simulink model "Fahrzeugmodell"  (R2020b)
settings: Solver=VariableStepAuto  StartTime=0.0  StopTime=inf  RelTol=1e-3
values from neighbouring files (symbols this model uses):
  a = 1.25    [Fahrdynamik.m]    (also in ZweiDFahranimation.m = 1.35)
  A_f = 1.6 + 0.00056*(m-765)    (= 1.933088)    [Fahrdynamik.m]
  aa = 0    [Fahrdynamik.m]
  b = []    [Bezier.m]    (also in Bezier1.m; Fahrdynamik.m = 1.35; TestenBezier.m; ZweiDFahranimation.m = 1.35)
  bb = 0.5    [Fahrdynamik.m]
  c1 = 52480    [Fahrdynamik.m]
  c2 = 88416    [Fahrdynamik.m]
  c_w = 0.34    [Fahrdynamik.m]
  f_r = 0.015    [Fahrdynamik.m]
  g = 9.81    [Fahrdynamik.m]
  Iz = 1992.54    [Fahrdynamik.m]
  m = 1359.8    [Fahrdynamik.m]
  roh = 1.225    [Fahrdynamik.m]
undefined symbols (not defined in the file or in its folder): DiscIntNeverNeededParam
libraries: simulink x10, simulink_extras x9, robotmobilelib x3, vrlib x1, sldrtlib x1, autolibshared x1
settings Model: SimulationMode=accelerator  PacingRate=0.100000  Creator=59258  LastModifiedBy=59258
settings SolverCC: AlgebraicLoopSolver=LineSearch
settings RTWCC: GenCodeOnly=on

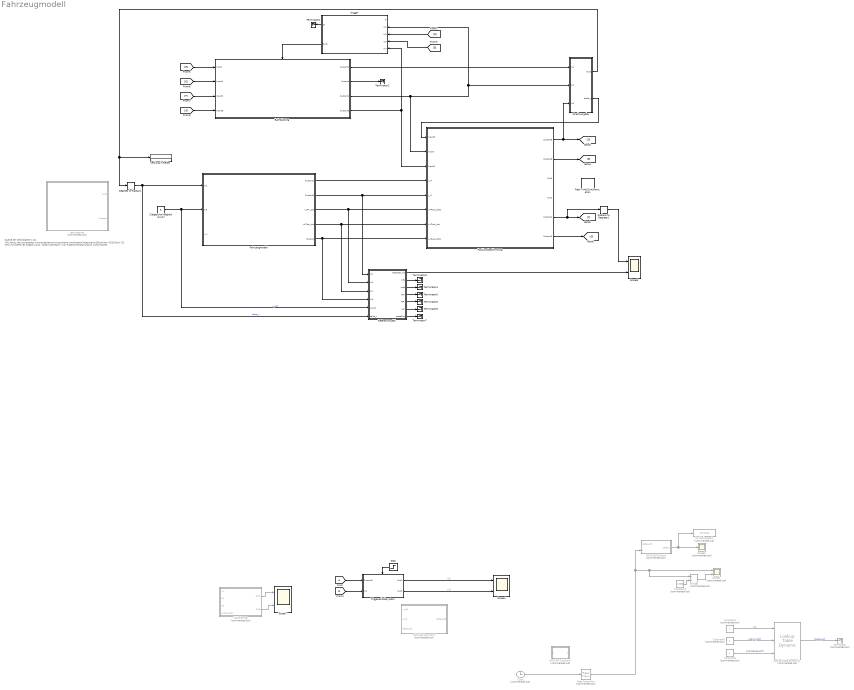
== system Fahrzeugmodell ==
  note: Quelle der Deckblättern:
      | [1] URL:https://en.nissanqatar.com/experience-nissan/news-and-events/latestnews/09-January-2019.html
      | [2] URL:Volvo/SPS
      | [3] Ziegler Julius, {Optimale Bahn- und Trajektorienplanung für Automoblie}
  Bahnplanung : Subsystem  TreatAsAtomicUnit=on  SystemSampleTime=111
      mask Display: image('Deckblatt.png'); % Use "Edit Image" on toolstrip to change.
  Clock : Clock  Commented=on
      settings: Decimation=1000
  Constant3 : Constant  Commented=on  Value=0.066
  Constant4 : Constant  Commented=on
  Constant5 : Constant  Commented=on
  Constant6 : Constant  Commented=on
  Degrees to Radians : simulink_extras/Transformations/Degrees to Radians
  Direktvorgabe : Subsystem
  Divide1 : Product  Commented=on  Inputs=*/
  Fahrzeugmodell : Subsystem  SystemSampleTime=0.5
      settings: MinAlgLoopOccurrences=on
      mask Display: image('Nissan Leaf.jpg'); % Use "Edit Image" on toolstrip to change.
  Kalibrierung : Subsystem  Commented=on  TreatAsAtomicUnit=on  SystemSampleTime=0.01
  Lenkung in Reifen : Display
  Lenkungsrad : Subsystem  Commented=on
  Lookup Table Dynamic1 : simulink/Lookup Tables/Lookup Table Dynamic  Commented=on  LookUpMeth=Use Input Above  OutDataType=fixdt('double')  OutScaling=[]  OutputDataTypeScalingMode=Specify via dialog  OutDataTypeStr=double  RndMeth=Convergent  DoSatur=off
  MATLAB Function : MATLAB Function  Commented=on  TreatAsAtomicUnit=on  SystemSampleTime=0.066
  MATLAB Function1 : MATLAB Function  Commented=on  TreatAsAtomicUnit=on
  MATLAB Function2 : MATLAB Function  Commented=on  TreatAsAtomicUnit=on
  Positionsbestimmung : Subsystem  SystemSampleTime=0.05
      mask Display: image('Volvo-testet-die-magnetische-Positionsbestimmung.jpg'); % Use "Edit Image" on toolstrip to change.
  Radians to Degrees1 : simulink_extras/Transformations/Radians to Degrees
  Rate Transition : RateTransition  Commented=on  OutPortSampleTime=0.066
  Real-Time Synchronization : sldrtlib/Real-Time Synchronization  SampleTime=0.1  MaxMissedTicks=30  ShowMissedTicks=off  YieldWhenWaiting=off
  Referenzmodell : Subsystem
  Scope1 : Scope  Commented=on  NumInputPorts=2
  Scope2 : Scope  Commented=on
  Scope3 : Scope  NumInputPorts=2
  Scope4 : Scope  NumInputPorts=2
  Scope7 : Scope  NumInputPorts=2
  Step : Step  Time=7.7  SampleTime=0
  Terminator : Terminator  Commented=on
  Terminator{1..8} (8 alike) : Terminator
  To Workspace1 : ToWorkspace  Commented=on  VariableName=simout1  SaveFormat=Timeseries  SampleTime=-1
  Trigger : Subsystem
  Triggered Subsystem : Subsystem  TreatAsAtomicUnit=on
  Zielgeschwindigkeit (km/h) : Constant  Value=5
  wires:
  Step/1 -> Triggered Subsystem/Trigger
  Triggered Subsystem/1(Out1) -> Scope4/1  "x_k"
  [A] -> Triggered Subsystem/1(Outport2)
  [B] -> Triggered Subsystem/2(In2)
  Triggered Subsystem/2(Out2) -> Scope4/2  "y_k"
  Kalibrierung/1(Out1) -> Scope7/1
  Kalibrierung/2(Out2) -> Scope7/2
  [F] -> Bahnplanung/3(Inport2)
  [G] -> Bahnplanung/4(Inport3)
  Degrees to Radians/1 -> Fahrzeugmodell/1(In1), Referenzmodell/6(delta_v)  "delta_v"
  Fahrzeugmodell/1(Outport1) -> Positionsbestimmung/4(x_M)
  Fahrzeugmodell/2(Outport2) -> Referenzmodell/1(In2), Positionsbestimmung/5(y_M)
  Fahrzeugmodell/3(x2=y_dot) -> Referenzmodell/2(In3), Positionsbestimmung/6(x4=psi_dot2)
  Positionsbestimmung/6(Outport2) -> [G]
  Bahnplanung/4(Outport3) -> Positionsbestimmung/3(Inport1), Trigger/5(In4)
  Rate Transition/1 -> MATLAB Function/2(t), Divide1/1, Scope1/1
  MATLAB Function/1(delta_v) -> To Workspace1/1, Scope2/1
  Clock/1 -> Rate Transition/1
  Constant3/1 -> Divide1/2
  Divide1/1 -> Scope1/2
  Positionsbestimmung/5(Outport1) -> [F], Radians to Degrees1/1
  Bahnplanung/3(Outport1) -> Trigger/2(In2), Direktvorgabe/2(In2), Positionsbestimmung/2(Inport)
  Radians to Degrees1/1 -> Scope3/1
  Fahrzeugmodell/4(x4=psi_dot) -> Referenzmodell/3(In4), Positionsbestimmung/7(x4=psi_dot)
  Positionsbestimmung/1(Outport5) -> Direktvorgabe/3(In3), [D]
  Positionsbestimmung/2(Outport6) -> [E]
  [D] -> Bahnplanung/1(Inport)
  [E] -> Bahnplanung/2(Inport1)
  Constant4/1 -> Lookup Table Dynamic1/1  "x_s"
  Lookup Table Dynamic1/1 -> Terminator/1  "kappa_soll"
  Constant5/1 -> Lookup Table Dynamic1/2  "Array[x_soll]"
  Constant6/1 -> Lookup Table Dynamic1/3  "Array[kappa_soll]"
  Fahrzeugmodell/5(Outport) -> Referenzmodell/4(In5), Positionsbestimmung/8(x4=psi_dot1)
  Bahnplanung/1(Outport2) -> Direktvorgabe/1(In1)
  Direktvorgabe/1(Out1) -> Degrees to Radians/1, Lenkung in Reifen/1
  Direktvorgabe/2(delta_v) -> Positionsbestimmung/1(Inport2)
  Zielgeschwindigkeit (km/h)/1 -> Referenzmodell/5(Input1), Fahrzeugmodell/2(In3)  "v_soll"
  Trigger/2(Out2) -> Bahnplanung/Enable
  Trigger/1(!Q) -> Terminator1/1
  Bahnplanung/2(Outport) -> Terminator2/1
  Referenzmodell/1(Degrees out) -> Scope3/2
  Referenzmodell/2(Info) -> Terminator3/1
  Referenzmodell/3(xdot) -> Terminator4/1
  Referenzmodell/4(FzF) -> Terminator5/1
  Referenzmodell/5(FzR) -> Terminator6/1
  Referenzmodell/7(stateDot) -> Terminator7/1
  Referenzmodell/6(psi) -> Terminator8/1
  [D] -> Trigger/3(In3)
  [E] -> Trigger/4(In5)

== system Fahrzeugmodell/Bahnplanung ==
  Inport : Inport
  Inport1 : Inport  Port=2
  Inport2 : Inport  Port=3
  Inport3 : Inport  Port=4
  Enable : EnablePort
  Constant : Constant  Value=0  VectorParams1D=off  SampleTime=-1
  Equal : RelationalOperator  Operator===  OutDataTypeStr=boolean  RndMeth=Simplest
  Scope : Scope
  Stop Simulation : Stop  Commented=on
  Subsystem : Subsystem
  Outport2 : Outport
  Outport : Outport  Port=2
  Outport1 : Outport  Port=3
  Outport3 : Outport  Port=4
  wires:
  Inport/1 -> Subsystem/1(Inport)  "x_s"
  Inport1/1 -> Subsystem/2(Inport1)  "y_s"
  Inport2/1 -> Subsystem/3(Inport2)  "psi_s"
  Inport3/1 -> Subsystem/4(Inport3)
  Subsystem/1(Outport1) -> Outport2/1
  Subsystem/2(Outport) -> Equal/1, Outport/1
  Subsystem/3(Outport2) -> Outport1/1
  Subsystem/4(Outport3) -> Outport3/1
  Constant/1 -> Equal/2
  Equal/1 -> Stop Simulation/1, Scope/1

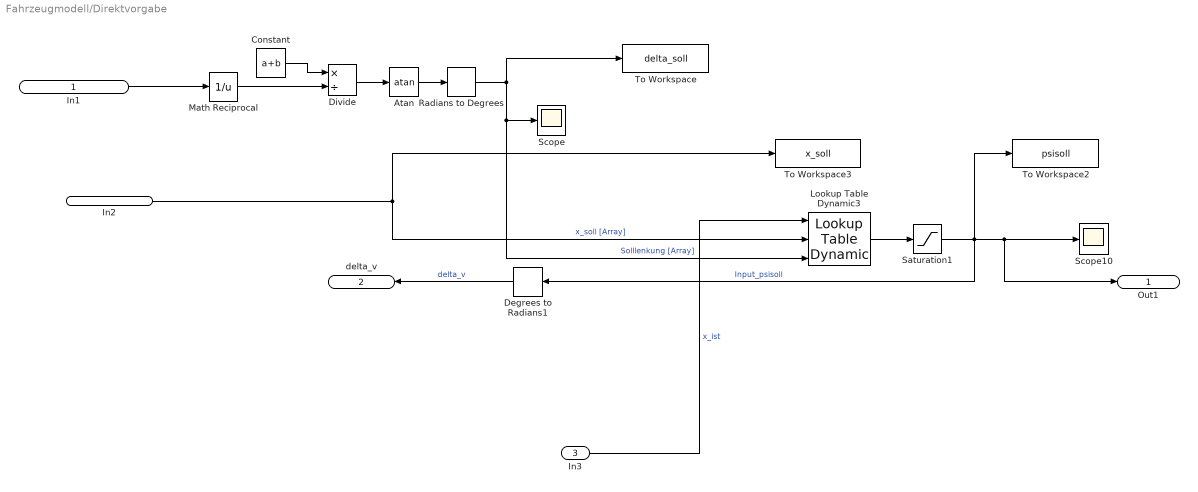
== system Fahrzeugmodell/Direktvorgabe ==
  In1 : Inport
  In2 : Inport  Port=2
  In3 : Inport  Port=3
  Atan : Trigonometry  Operator=atan
  Constant : Constant  Value=a+b
  Degrees to Radians1 : simulink_extras/Transformations/Degrees to Radians
  Divide : Product  Inputs=*/  RndMeth=Zero  SaturateOnIntegerOverflow=on
  Lookup Table Dynamic3 : simulink/Lookup Tables/Lookup Table Dynamic  LookUpMeth=Use Input Nearest  OutDataType=fixdt('double')  OutScaling=[]  OutputDataTypeScalingMode=Specify via dialog  OutDataTypeStr=double  RndMeth=Nearest  DoSatur=off
  Math Reciprocal : Math  Operator=reciprocal  SignedPower=on  SaturateOnIntegerOverflow=on
  Radians to Degrees : simulink_extras/Transformations/Radians to Degrees
  Saturation1 : Saturate  UpperLimit=24.46  LowerLimit=-24.46
  Scope : Scope
  Scope10 : Scope
  To Workspace : ToWorkspace  VariableName=delta_soll  SaveFormat=Timeseries  SampleTime=-1
  To Workspace2 : ToWorkspace  VariableName=psisoll  SaveFormat=Timeseries  SampleTime=-1
  To Workspace3 : ToWorkspace  VariableName=x_soll  SaveFormat=Timeseries  SampleTime=-1
  Out1 : Outport
  delta_v : Outport  Port=2
  wires:
  Math Reciprocal/1 -> Divide/2
  Saturation1/1 -> Degrees to Radians1/1, Out1/1, Scope10/1, To Workspace2/1  "Input_psisoll"
  Atan/1 -> Radians to Degrees/1
  Divide/1 -> Atan/1
  Lookup Table Dynamic3/1 -> Saturation1/1
  Radians to Degrees/1 -> Lookup Table Dynamic3/3, Scope/1, To Workspace/1  "Solllenkung [Array]"
  In3/1 -> Lookup Table Dynamic3/1  "x_ist"
  In2/1 -> Lookup Table Dynamic3/2, To Workspace3/1  "x_soll [Array]"
  Constant/1 -> Divide/1
  In1/1 -> Math Reciprocal/1
  Degrees to Radians1/1 -> delta_v/1  "delta_v"

== system Fahrzeugmodell/Fahrzeugmodell ==
  In1 : Inport
  In3 : Inport  Port=2
  v_x : Inport  Port=3
  Laengsdynamik : Subsystem
  Querdynamik : Subsystem
  Scope : Scope  NumInputPorts=5
  Scope1 : Scope  NumInputPorts=2
  physikalische Koordinate : Subsystem
  Outport1 : Outport
  Outport2 : Outport  Port=2
  x2=y_dot : Outport  Port=3
  x4=psi_dot : Outport  Port=4
  Outport : Outport  Port=5
  wires:
  Querdynamik/2(x2=y_dot) -> Scope/2, x2=y_dot/1, Laengsdynamik/2(Inport)
  Querdynamik/3(x3=psi) -> Scope/3
  Querdynamik/1(x1=y) -> Scope/1
  Querdynamik/5(Outport) -> Scope/5
  Querdynamik/4(x4=psi_dot) -> Laengsdynamik/3(Inport1), x4=psi_dot/1, Scope/4, physikalische Koordinate/2(x4=psi_dot)
  In3/1 -> Laengsdynamik/1(In1)
  physikalische Koordinate/1(x_Koordinate des Modells um Antenne) -> Outport1/1
  In1/1 -> Querdynamik/1(In1)
  physikalische Koordinate/2(Outport2) -> Outport2/1
  Laengsdynamik/2(Out1) -> Scope1/2
  Laengsdynamik/1(v_x) -> Outport/1, Scope1/1, physikalische Koordinate/1(v_x), Querdynamik/2(v_x)

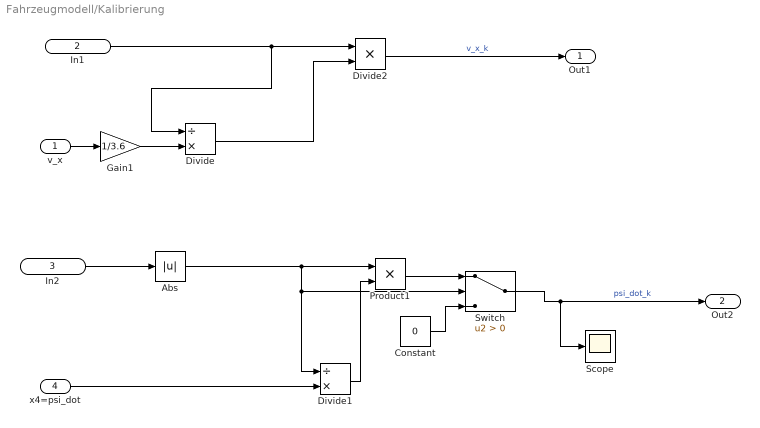
== system Fahrzeugmodell/Kalibrierung ==
  v_x : Inport
  In1 : Inport  Port=2
  In2 : Inport  Port=3
  x4=psi_dot : Inport  Port=4
  Abs : Abs
  Constant : Constant  Value=0
  Divide : Product  Inputs=/*
  Divide1 : Product  Inputs=/*
  Divide2 : Product  Inputs=**
  Gain1 : Gain  Gain=1/3.6
  Product1 : Product
  Scope : Scope
  Switch : Switch  Criteria=u2 > Threshold
  Out1 : Outport
  Out2 : Outport  Port=2
  wires:
  Divide2/1 -> Out1/1  "v_x_k"
  Divide/1 -> Divide2/2
  x4=psi_dot/1 -> Divide1/2
  Product1/1 -> Switch/1
  In2/1 -> Abs/1
  In1/1 -> Divide2/1, Divide/1
  Gain1/1 -> Divide/2
  v_x/1 -> Gain1/1
  Divide1/1 -> Product1/2
  Constant/1 -> Switch/3
  Abs/1 -> Divide1/1, Switch/2, Product1/1
  Switch/1 -> Out2/1, Scope/1  "psi_dot_k"

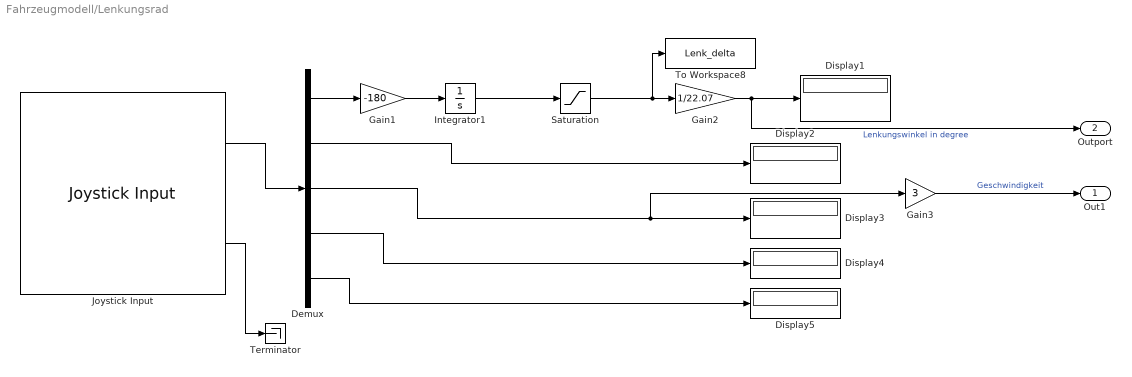
== system Fahrzeugmodell/Lenkungsrad ==
  Demux : Demux  Outputs=5
  Display{1..5} (5 alike) : Display
  Gain1 : Gain  Gain=-180
  Gain2 : Gain  Gain=1/22.07
  Gain3 : Gain  Gain=3
  Integrator1 : Integrator  InitialCondition=0.001
  Joystick Input : vrlib/Joystick Input  joyid=1  adjustports=on  forcefeed=off
  Saturation : Saturate  UpperLimit=540  LowerLimit=-540
  Terminator : Terminator
  To Workspace8 : ToWorkspace  VariableName=Lenk_delta  SaveFormat=Timeseries  SampleTime=-1
  Out1 : Outport
  Outport : Outport  Port=2
  wires:
  Joystick Input/1 -> Demux/1
  Saturation/1 -> To Workspace8/1, Gain2/1
  Gain2/1 -> Outport/1, Display1/1  "Lenkungswinkel in degree"
  Demux/3 -> Gain3/1, Display3/1
  Integrator1/1 -> Saturation/1
  Joystick Input/2 -> Terminator/1
  Demux/2 -> Display2/1
  Demux/1 -> Gain1/1
  Demux/4 -> Display4/1
  Gain1/1 -> Integrator1/1
  Demux/5 -> Display5/1
  Gain3/1 -> Out1/1  "Geschwindigkeit"

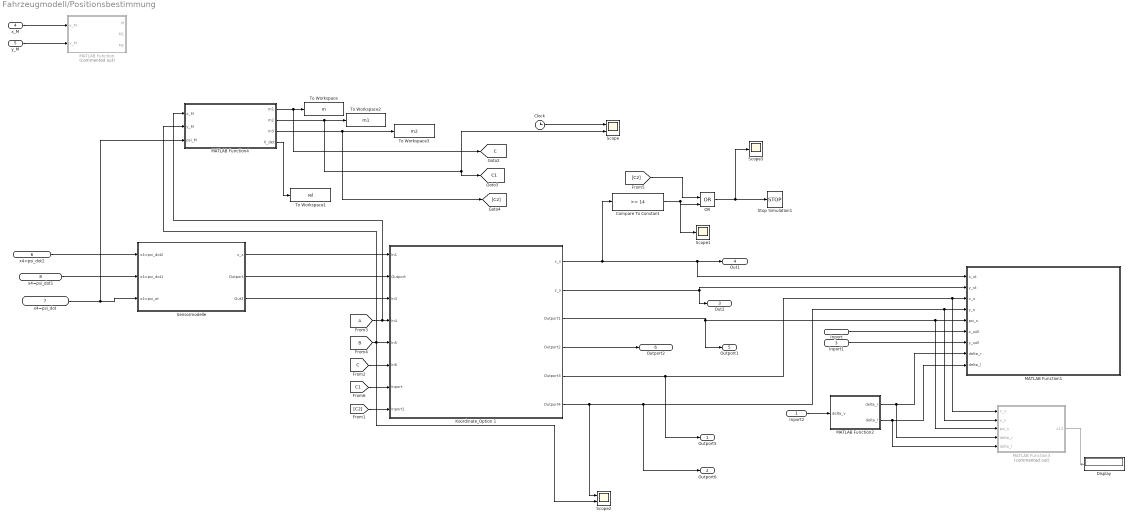
== system Fahrzeugmodell/Positionsbestimmung ==
  Inport2 : Inport
  Inport : Inport  Port=2
  Inport1 : Inport  Port=3
  x_M : Inport  Port=4
  y_M : Inport  Port=5
  x4=psi_dot2 : Inport  Port=6
  x4=psi_dot : Inport  Port=7
  x4=psi_dot1 : Inport  Port=8
  Clock : Clock
  Compare To Constant : simulink/Logic and Bit Operations/Compare To Constant  relop=>=  const=14  OutDataTypeStr=boolean
  Display : Display
  Koordinate_Option 1 : Subsystem
  MATLAB Function : MATLAB Function  Commented=on  TreatAsAtomicUnit=on  SystemSampleTime=0.01
  MATLAB Function1 : MATLAB Function  TreatAsAtomicUnit=on  SystemSampleTime=0.2
  MATLAB Function2 : MATLAB Function  TreatAsAtomicUnit=on
  MATLAB Function3 : MATLAB Function  Commented=on  TreatAsAtomicUnit=on  SystemSampleTime=0.5
  MATLAB Function4 : MATLAB Function  TreatAsAtomicUnit=on
  OR : Logic  Operator=OR  IconShape=distinctive  AllPortsSameDT=off  OutDataTypeStr=boolean
  Scope : Scope  NumInputPorts=2
  Scope1 : Scope
  Scope2 : Scope  NumInputPorts=2
  Scope3 : Scope
  Sensormodelle : Subsystem
  Stop Simulation1 : Stop
  To Workspace : ToWorkspace  VariableName=m  SaveFormat=Timeseries  SampleTime=-1
  To Workspace1 : ToWorkspace  VariableName=rel  SaveFormat=Timeseries  SampleTime=-1
  To Workspace2 : ToWorkspace  VariableName=m1  SaveFormat=Timeseries  SampleTime=-1
  To Workspace3 : ToWorkspace  VariableName=m2  SaveFormat=Timeseries  SampleTime=-1
  Outport5 : Outport
  Outport6 : Outport  Port=2
  Out2 : Outport  Port=3
  Out1 : Outport  Port=4
  Outport1 : Outport  Port=5
  Outport2 : Outport  Port=6
  tag scope: C1=global, C=global
  wires:
  Sensormodelle/2(Outport) -> Koordinate_Option 1/2(Outport)
  [A] -> MATLAB Function4/1(x_M), Koordinate_Option 1/4(In4)
  [C] -> Koordinate_Option 1/6(In6)
  Sensormodelle/1(v_x) -> Koordinate_Option 1/1(In1)
  Sensormodelle/3(Out3) -> Koordinate_Option 1/3(In3)
  Koordinate_Option 1/4(Outport2) -> Outport2/1
  x_M/1 -> MATLAB Function/1(x_M)
  [B] -> Scope2/2, MATLAB Function4/2(y_M), Koordinate_Option 1/5(In5)
  Koordinate_Option 1/1(x_s) -> MATLAB Function1/1(x_st), Out1/1, Compare To Constant/1
  x4=psi_dot1/1 -> Sensormodelle/2(x4=psi_dot1)
  Koordinate_Option 1/3(Outport1) -> Outport1/1, MATLAB Function3/3(psi_s), MATLAB Function1/5(psi_s)
  Koordinate_Option 1/2(y_s) -> MATLAB Function1/2(y_st), Out2/1
  x4=psi_dot/1 -> MATLAB Function4/3(psi_M), Sensormodelle/3(x4=psi_ot)
  x4=psi_dot2/1 -> Sensormodelle/1(x4=psi_dot2)
  [C1] -> Koordinate_Option 1/7(Inport)
  [C2] -> Koordinate_Option 1/8(Inport1)
  Clock/1 -> Scope/1
  Compare To Constant/1 -> Scope1/1, OR/2
  Inport/1 -> MATLAB Function1/6(x_soll)
  Inport1/1 -> MATLAB Function1/7(y_soll)
  OR/1 -> Scope3/1, Stop Simulation1/1
  Koordinate_Option 1/6(Outport4) -> Scope2/1, Outport6/1, MATLAB Function3/2(y_s), MATLAB Function1/4(y_s)
  Inport2/1 -> MATLAB Function2/1(delta_v)
  MATLAB Function2/1(delta_r) -> MATLAB Function3/4(delta_r), MATLAB Function1/8(delta_r)
  MATLAB Function2/2(delta_l) -> MATLAB Function3/5(delta_l), MATLAB Function1/9(delta_l)
  Koordinate_Option 1/5(Outport3) -> Outport5/1, MATLAB Function3/1(x_s), MATLAB Function1/3(x_s)
  MATLAB Function3/1(x12) -> Display/1
  [C2] -> OR/1
  y_M/1 -> MATLAB Function/2(y_M)
  MATLAB Function4/1(m1) -> [C], To Workspace/1
  MATLAB Function4/4(X_det) -> To Workspace1/1
  MATLAB Function4/2(m2) -> Scope/2, [C1], To Workspace2/1
  MATLAB Function4/3(m3) -> [C2], To Workspace3/1

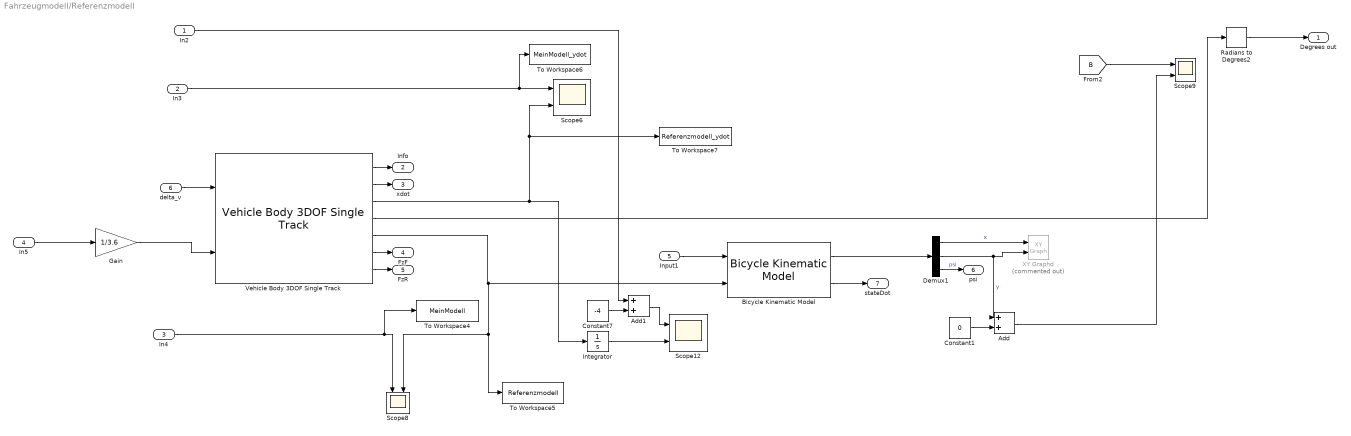
== system Fahrzeugmodell/Referenzmodell ==
  In2 : Inport
  In3 : Inport  Port=2
  In4 : Inport  Port=3
  In5 : Inport  Port=4
  Input1 : Inport  Port=5
  delta_v : Inport  Port=6
  Add : Sum
  Add1 : Sum
  Bicycle Kinematic Model : robotmobilelib/Bicycle Kinematic Model  VehicleInputs=Vehicle Speed & Heading Angular Velocity  WheelBase=1  VehicleSpeedRange=[-inf inf]  MaxSteeringAngle=pi/4  InitialState=[0; 0; 0]  SimulateUsing=Interpreted execution
      settings: SourceProductBaseCode=RO
  Constant1 : Constant  Value=0
  Constant7 : Constant  Value=-4
  Demux1 : Demux  Outputs=3
  Gain : Gain  Gain=1/3.6
  Integrator : Integrator
  Radians to Degrees2 : simulink_extras/Transformations/Radians to Degrees
  Scope{6,8..9,12} (4 alike) : Scope  NumInputPorts=2
  To Workspace4 : ToWorkspace  VariableName=MeinModell  SaveFormat=Timeseries  SampleTime=-1
  To Workspace5 : ToWorkspace  VariableName=Referenzmodell  SaveFormat=Timeseries  SampleTime=-1
  To Workspace6 : ToWorkspace  VariableName=MeinModell_ydot  SaveFormat=Timeseries  SampleTime=-1
  To Workspace7 : ToWorkspace  VariableName=Referenzmodell_ydot  SaveFormat=Timeseries  SampleTime=-1
  Vehicle Body 3DOF Single Track : autolibshared/Vehicle Body 3DOF Single Track  trackMode=Single (bicycle)  inputMode=External longitudinal velocity  frontSteerMode=on  rearSteerMode=off  windMode=off  muMode=off  extFMode=off  extMMode=off  htchFMode=off  htchMMode=off  extXo=off  extpsio=off  extxdoto=off  extro=off  extYo=off  extTamb=off  extydoto=off  aMode=2  NF=2  NR=2  m=1359.8  a=1.25  b=1.35  h=0.35  dh=1  hh=0.2  X_o=0  xdot_o=0  CalphaMode=off  sigmaMode=on  d=0  hl=0  w=[1.4,1.4]  Cy_f=52480  Cy_r=88416  sigma_f=.1  sigma_r=.1  alpha_f_brk=[-.1 .1]  Cy_f_data=[-9e3 9e3]  alpha_r_brk=[-.1 .1]  Cy_r_data=[-9e3 9e3]  Y_o=0  ydot_o=0  Izz=1992.54  psi_o=0  r_o=0  Af=1.9331  Cd=.34  Cl=.1  Cpm=.1  beta_w=[0:0.01:0.3]  Cs=[0:0.03:0.9]  Cym=[0:0.01:0.3]  Pabs=101325  Tair=273  g=9.81  mu=1  xdot_tol=.01  Fznom=5000  Fxtire_sat=7e4  Fytire_sat=7e4  longOff=0  latOff=0  vertOff=0  wrapAng=off
      settings: SourceProductBaseCode=PW,MT,UV,VE,VP
  XY Graphd : simulink/Sinks/XY Graph  Commented=on  xmin=-3  xmax=20  ymin=-3  ymax=20  st=0.1
  Degrees out : Outport
  Info : Outport  Port=2
  xdot : Outport  Port=3
  FzF : Outport  Port=4
  FzR : Outport  Port=5
  psi : Outport  Port=6
  stateDot : Outport  Port=7
  wires:
  delta_v/1 -> Vehicle Body 3DOF Single Track/1
  Add1/1 -> Scope12/1
  Vehicle Body 3DOF Single Track/3 -> Scope6/2, To Workspace7/1, Integrator/1
  In4/1 -> To Workspace4/1, Scope8/1
  Vehicle Body 3DOF Single Track/5 -> Scope8/2, To Workspace5/1, Bicycle Kinematic Model/2
  Vehicle Body 3DOF Single Track/4 -> Radians to Degrees2/1
  Demux1/2 -> XY Graphd/2, Add/1  "y"
  In3/1 -> To Workspace6/1, Scope6/1
  Add/1 -> Scope9/2
  Vehicle Body 3DOF Single Track/2 -> xdot/1
  Constant1/1 -> Add/2
  Demux1/1 -> XY Graphd/1  "x"
  Bicycle Kinematic Model/1 -> Demux1/1
  Vehicle Body 3DOF Single Track/7 -> FzR/1
  Integrator/1 -> Scope12/2
  Vehicle Body 3DOF Single Track/1 -> Info/1
  Constant7/1 -> Add1/2
  [B] -> Scope9/1
  Gain/1 -> Vehicle Body 3DOF Single Track/2
  Demux1/3 -> psi/1  "psi"
  In5/1 -> Gain/1
  In2/1 -> Add1/1
  Vehicle Body 3DOF Single Track/6 -> FzF/1
  Radians to Degrees2/1 -> Degrees out/1
  Input1/1 -> Bicycle Kinematic Model/1
  Bicycle Kinematic Model/2 -> stateDot/1

== system Fahrzeugmodell/Trigger ==
  R : Inport
  In2 : Inport  Port=2
  In3 : Inport  Port=3
  In5 : Inport  Port=4
  In4 : Inport  Port=5
  Subsystem1 : Subsystem
  Subsystem2 : Subsystem
  !Q : Outport
  Out2 : Outport  Port=2
  wires:
  Subsystem1/1(y) -> Subsystem2/2(Ja/Nein)
  Subsystem2/1(!Q) -> !Q/1
  In2/1 -> Subsystem1/2(In2)
  R/1 -> Subsystem2/1(R)
  In3/1 -> Subsystem1/1(In1)
  Subsystem2/2(Out2) -> Out2/1  "Ja/nein"
  In4/1 -> Subsystem1/3(In3)
  In5/1 -> Subsystem1/4(In4)

== system Fahrzeugmodell/Triggered Subsystem ==
  Outport2 : Inport
  In2 : Inport  Port=2
  Trigger : TriggerPort  VariantControl=Variant
  Out1 : Outport
  Out2 : Outport  Port=2
  wires:
  Outport2/1 -> Out1/1
  In2/1 -> Out2/1

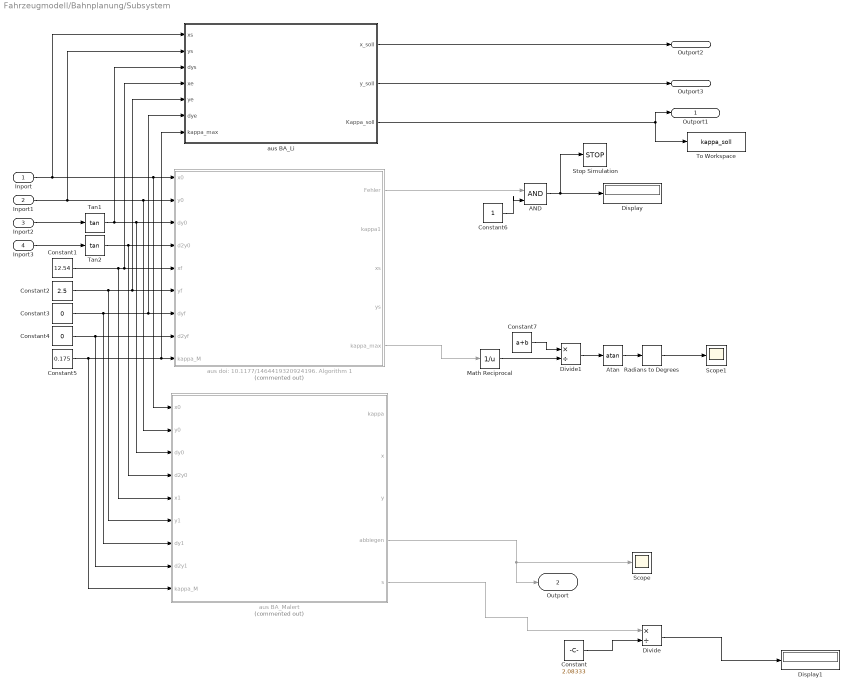
== system Fahrzeugmodell/Bahnplanung/Subsystem ==
  Inport : Inport
  Inport1 : Inport  Port=2
  Inport2 : Inport  Port=3
  Inport3 : Inport  Port=4
  AND : Logic  IconShape=distinctive  AllPortsSameDT=off  OutDataTypeStr=boolean
  Atan : Trigonometry  Operator=atan
  Constant : Constant  Value=2.08333
  Constant1 : Constant  Value=12.54
  Constant2 : Constant  Value=2.5
  Constant3 : Constant  Value=0
  Constant4 : Constant  Value=0
  Constant5 : Constant  Value=0.175
  Constant6 : Constant
  Constant7 : Constant  Value=a+b
  Display : Display
  Display1 : Display
  Divide : Product  Inputs=*/
  Divide1 : Product  Inputs=*/  RndMeth=Zero  SaturateOnIntegerOverflow=on
  Math Reciprocal : Math  Operator=reciprocal  SignedPower=on  SaturateOnIntegerOverflow=on
  Radians to Degrees : simulink_extras/Transformations/Radians to Degrees
  Scope : Scope
  Scope1 : Scope
  Stop Simulation : Stop
  Tan1 : Trigonometry  Operator=tan
  Tan2 : Trigonometry  Operator=tan
  To Workspace : ToWorkspace  VariableName=kappa_soll  SaveFormat=Timeseries  SampleTime=-1
  aus BA_Li : MATLAB Function  TreatAsAtomicUnit=on
  aus BA_Malert : MATLAB Function  Commented=on  TreatAsAtomicUnit=on
  aus doi: 10.1177/1464419320924196. Algorithm 1 : MATLAB Function  Commented=on  TreatAsAtomicUnit=on
  Outport1 : Outport
  Outport : Outport  Port=2
  Outport2 : Outport  Port=3
  Outport3 : Outport  Port=4
  wires:
  Constant1/1 -> aus BA_Li/4(xe), aus doi: 10.1177/1464419320924196. Algorithm 1/5(xf), aus BA_Malert/5(x1)
  Constant2/1 -> aus BA_Malert/6(y1), aus BA_Li/5(ye), aus doi: 10.1177/1464419320924196. Algorithm 1/6(yf)
  Constant4/1 -> aus BA_Malert/8(d2y1), aus doi: 10.1177/1464419320924196. Algorithm 1/8(d2yf)
  Constant3/1 -> aus BA_Malert/7(dy1), aus BA_Li/6(dye), aus doi: 10.1177/1464419320924196. Algorithm 1/7(dyf)
  Inport1/1 -> aus BA_Li/2(ys), aus BA_Malert/2(y0), aus doi: 10.1177/1464419320924196. Algorithm 1/2(y0)
  Constant5/1 -> aus BA_Malert/9(kappa_M), aus BA_Li/7(kappa_max), aus doi: 10.1177/1464419320924196. Algorithm 1/9(kappa_M)
  aus BA_Malert/4(abbiegen) -> Outport/1, Scope/1
  aus BA_Malert/5(s) -> Divide/1
  Constant/1 -> Divide/2
  Divide/1 -> Display1/1
  Tan1/1 -> aus BA_Li/3(dys), aus BA_Malert/3(dy0), aus doi: 10.1177/1464419320924196. Algorithm 1/3(dy0)
  Tan2/1 -> aus BA_Malert/4(d2y0), aus doi: 10.1177/1464419320924196. Algorithm 1/4(d2y0)
  Inport2/1 -> Tan1/1
  Inport3/1 -> Tan2/1
  Constant6/1 -> AND/2
  aus doi: 10.1177/1464419320924196. Algorithm 1/1(Fehler) -> AND/1
  AND/1 -> Display/1, Stop Simulation/1
  Atan/1 -> Radians to Degrees/1
  Constant7/1 -> Divide1/1
  Divide1/1 -> Atan/1
  Math Reciprocal/1 -> Divide1/2
  aus doi: 10.1177/1464419320924196. Algorithm 1/5(kappa_max) -> Math Reciprocal/1
  Radians to Degrees/1 -> Scope1/1
  aus BA_Li/3(Kappa_soll) -> To Workspace/1, Outport1/1
  aus BA_Li/1(x_soll) -> Outport2/1
  aus BA_Li/2(y_soll) -> Outport3/1
  Inport/1 -> aus BA_Li/1(xs), aus BA_Malert/1(x0), aus doi: 10.1177/1464419320924196. Algorithm 1/1(x0)

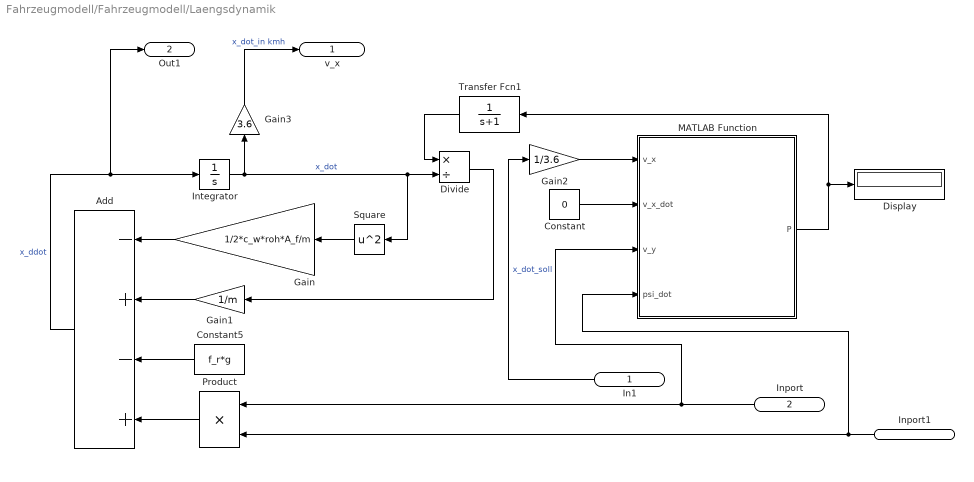
== system Fahrzeugmodell/Fahrzeugmodell/Laengsdynamik ==
  In1 : Inport
  Inport : Inport  Port=2
  Inport1 : Inport  Port=3
  Add : Sum  Inputs=-+-+
  Constant : Constant  Value=0
  Constant5 : Constant  Value=f_r*g
  Display : Display
  Divide : Product  Inputs=*/
  Gain : Gain  Gain=1/2*c_w*roh*A_f/m
  Gain1 : Gain  Gain=1/m
  Gain2 : Gain  Gain=1/3.6
  Gain3 : Gain  Gain=3.6
  Integrator : Integrator  InitialCondition=0.01
  MATLAB Function : MATLAB Function  TreatAsAtomicUnit=on
  Product : Product
  Square : Math  Operator=square  SaturateOnIntegerOverflow=on
  Transfer Fcn1 : TransferFcn  Denominator=[1 1]
  v_x : Outport
  Out1 : Outport  Port=2
  wires:
  Gain1/1 -> Add/2
  Transfer Fcn1/1 -> Divide/1
  Square/1 -> Gain/1
  Integrator/1 -> Divide/2, Square/1, Gain3/1  "x_dot"
  Constant5/1 -> Add/3
  Add/1 -> Out1/1, Integrator/1  "x_ddot"
  Gain/1 -> Add/1
  Divide/1 -> Gain1/1
  MATLAB Function/1(P) -> Display/1, Transfer Fcn1/1
  Gain2/1 -> MATLAB Function/1(v_x)
  In1/1 -> Gain2/1  "x_dot_soll"
  Gain3/1 -> v_x/1  "x_dot_in kmh"
  Product/1 -> Add/4
  Inport/1 -> MATLAB Function/3(v_y), Product/1
  Inport1/1 -> Product/2, MATLAB Function/4(psi_dot)
  Constant/1 -> MATLAB Function/2(v_x_dot)

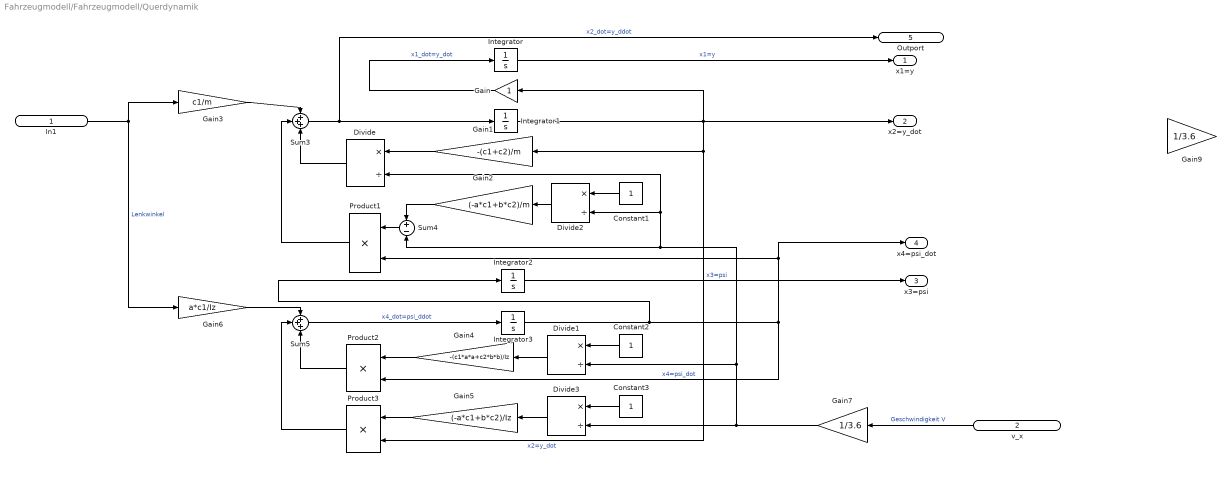
== system Fahrzeugmodell/Fahrzeugmodell/Querdynamik ==
  In1 : Inport
  v_x : Inport  Port=2
  Constant1 : Constant
  Constant2 : Constant
  Constant3 : Constant
  Divide{,1..3} (4 alike) : Product  Inputs=*/
  Gain : Gain
  Gain1 : Gain  Gain=-(c1+c2)/m
  Gain2 : Gain  Gain=(-a*c1+b*c2)/m
  Gain3 : Gain  Gain=c1/m
  Gain4 : Gain  Gain=-(c1*a*a+c2*b*b)/Iz
  Gain5 : Gain  Gain=(-a*c1+b*c2)/Iz
  Gain6 : Gain  Gain=a*c1/Iz
  Gain7 : Gain  Gain=1/3.6
  Gain9 : Gain  Gain=1/3.6
  Integrator{,1..3} (4 alike) : Integrator
  Product1 : Product
  Product2 : Product
  Product3 : Product
  Sum3 : Sum  Inputs=+++
  Sum4 : Sum  Inputs=+-
  Sum5 : Sum  Inputs=+++
  x1=y : Outport
  x2=y_dot : Outport  Port=2
  x3=psi : Outport  Port=3
  x4=psi_dot : Outport  Port=4
  Outport : Outport  Port=5
  wires:
  Gain/1 -> Integrator/1  "x1_dot=y_dot"
  Integrator3/1 -> Product2/2, Product1/2, x4=psi_dot/1, Integrator2/1  "x4=psi_dot"
  Gain1/1 -> Divide/1
  Sum3/1 -> Outport/1, Integrator1/1  "x2_dot=y_ddot"
  Product3/1 -> Sum5/2
  Gain6/1 -> Sum5/1
  v_x/1 -> Gain7/1  "Geschwindigkeit V"
  Sum4/1 -> Product1/1
  Gain2/1 -> Sum4/1
  Product1/1 -> Sum3/2
  Gain5/1 -> Product3/1
  Integrator1/1 -> x2=y_dot/1, Gain/1, Product3/2, Gain1/1  "x2=y_dot"
  In1/1 -> Gain6/1, Gain3/1  "Lenkwinkel"
  Constant1/1 -> Divide2/1
  Product2/1 -> Sum5/3
  Constant2/1 -> Divide1/1
  Divide3/1 -> Gain5/1
  Divide/1 -> Sum3/3
  Gain4/1 -> Product2/1
  Divide1/1 -> Gain4/1
  Sum5/1 -> Integrator3/1  "x4_dot=psi_ddot"
  Constant3/1 -> Divide3/1
  Integrator2/1 -> x3=psi/1  "x3=psi"
  Gain3/1 -> Sum3/1
  Divide2/1 -> Gain2/1
  Integrator/1 -> x1=y/1  "x1=y"
  Gain7/1 -> Divide3/2, Divide/2, Divide2/2, Sum4/2, Divide1/2

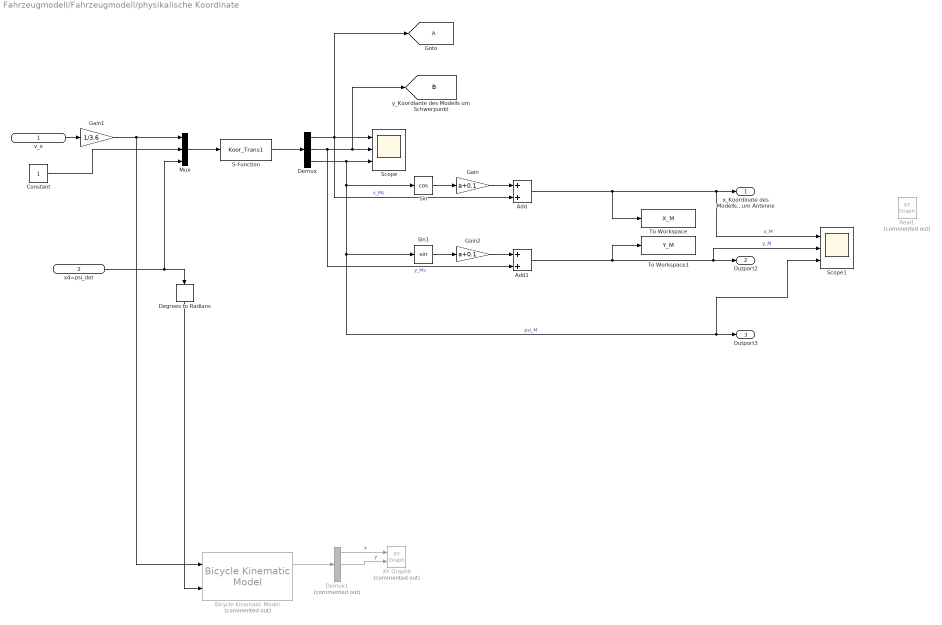
== system Fahrzeugmodell/Fahrzeugmodell/physikalische Koordinate ==
  v_x : Inport
  x4=psi_dot : Inport  Port=2
  Add : Sum
  Add1 : Sum
  Bicycle Kinematic Model : robotmobilelib/Bicycle Kinematic Model  Commented=on  VehicleInputs=Vehicle Speed & Heading Angular Velocity  WheelBase=1  VehicleSpeedRange=[-inf inf]  MaxSteeringAngle=pi/4  InitialState=[0; 0; 0]  SimulateUsing=Interpreted execution
      settings: SourceProductBaseCode=RO
  Constant : Constant
  Degrees to Radians : simulink_extras/Transformations/Degrees to Radians
  Demux : Demux  Outputs=3
  Demux1 : Demux  Commented=on  Outputs=3
  Gain : Gain  Gain=a+0.1
  Gain1 : Gain  Gain=1/3.6
  Gain2 : Gain  Gain=a+0.1
  Mux : Mux  Inputs=3
  Real1 : simulink/Sinks/XY Graph  Commented=on  xmin=0  xmax=40  ymin=0  ymax=15  st=0.1
  S-Function : S-Function  FunctionName=Koor_Trans1  Parameters=aa,bb  SFunctionDeploymentMode=off  EnableBusSupport=off
  Scope : Scope  NumInputPorts=3
  Scope1 : Scope  NumInputPorts=3
  Sin : Trigonometry  Operator=cos
  Sin1 : Trigonometry
  To Workspace : ToWorkspace  VariableName=X_M  SampleTime=-1
      settings: Save2DSignal=2-D array (concatenate along first dimension)
  To Workspace1 : ToWorkspace  VariableName=Y_M  SampleTime=-1
      settings: Save2DSignal=2-D array (concatenate along first dimension)
  XY Graphb : simulink/Sinks/XY Graph  Commented=on  xmin=-1  xmax=20  ymin=-1  ymax=3  st=0.1
  x_Koordinate des Modells um Antenne : Outport
  Outport2 : Outport  Port=2
  Outport3 : Outport  Port=3
  tag scope: A=global, B=global
  wires:
  Degrees to Radians/1 -> Bicycle Kinematic Model/2
  Demux1/2 -> XY Graphb/2  "y"
  Demux1/1 -> XY Graphb/1  "x"
  Constant/1 -> Mux/2
  Bicycle Kinematic Model/1 -> Demux1/1
  x4=psi_dot/1 -> Degrees to Radians/1, Mux/3
  v_x/1 -> Gain1/1
  Demux/3 -> Scope1/3, Outport3/1, Sin1/1, Sin/1, Scope/3  "psi_M"
  S-Function/1 -> Demux/1
  Mux/1 -> S-Function/1
  Gain1/1 -> Mux/1, Bicycle Kinematic Model/1
  Demux/2 -> Add1/2, [B], Scope/2  "y_Ms"
  Gain/1 -> Add/1
  Sin/1 -> Gain/1
  Add/1 -> To Workspace/1, Scope1/1, x_Koordinate des Modells um Antenne/1  "x_M"
  Add1/1 -> Scope1/2, Outport2/1, To Workspace1/1  "y_M"
  Sin1/1 -> Gain2/1
  Gain2/1 -> Add1/1
  Demux/1 -> [A], Add/2, Scope/1  "x_Ms"

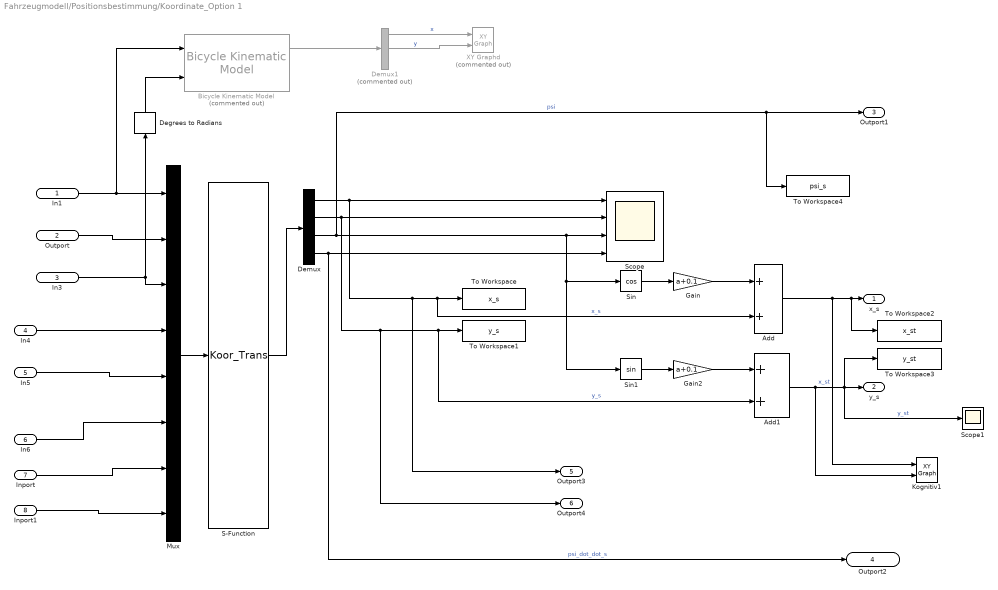
== system Fahrzeugmodell/Positionsbestimmung/Koordinate_Option 1 ==
  In1 : Inport
  Outport : Inport  Port=2
  In3 : Inport  Port=3
  In4 : Inport  Port=4
  In5 : Inport  Port=5
  In6 : Inport  Port=6
  Inport : Inport  Port=7
  Inport1 : Inport  Port=8
  Add : Sum
  Add1 : Sum
  Bicycle Kinematic Model : robotmobilelib/Bicycle Kinematic Model  Commented=on  VehicleInputs=Vehicle Speed & Heading Angular Velocity  WheelBase=1  VehicleSpeedRange=[-inf inf]  MaxSteeringAngle=pi/4  InitialState=[0; 0; 0]  SimulateUsing=Interpreted execution
      settings: SourceProductBaseCode=RO
  Degrees to Radians : simulink_extras/Transformations/Degrees to Radians
  Demux : Demux
  Demux1 : Demux  Commented=on  Outputs=3
  Gain : Gain  Gain=a+0.1
  Gain2 : Gain  Gain=a+0.1
  Kognitiv1 : simulink/Sinks/XY Graph  xmin=0  xmax=20  ymin=0  ymax=5  st=0.1
  Mux : Mux  Inputs=8
  S-Function : S-Function  FunctionName=Koor_Trans  Parameters=aa, bb  SFunctionDeploymentMode=off  EnableBusSupport=off
  Scope : Scope  NumInputPorts=4
  Scope1 : Scope
  Sin : Trigonometry  Operator=cos
  Sin1 : Trigonometry
  To Workspace : ToWorkspace  VariableName=x_s  SampleTime=-1
      settings: Save2DSignal=2-D array (concatenate along first dimension)
  To Workspace1 : ToWorkspace  VariableName=y_s  SampleTime=-1
      settings: Save2DSignal=2-D array (concatenate along first dimension)
  To Workspace2 : ToWorkspace  VariableName=x_st  SaveFormat=Timeseries  SampleTime=-1
  To Workspace3 : ToWorkspace  VariableName=y_st  SaveFormat=Timeseries  SampleTime=-1
  To Workspace4 : ToWorkspace  VariableName=psi_s  SaveFormat=Timeseries  SampleTime=-1
  XY Graphd : simulink/Sinks/XY Graph  Commented=on  xmin=-3  xmax=20  ymin=-1  ymax=3  st=0.1
  x_s : Outport
  y_s : Outport  Port=2
  Outport1 : Outport  Port=3
  Outport2 : Outport  Port=4
  Outport3 : Outport  Port=5
  Outport4 : Outport  Port=6
  wires:
  Mux/1 -> S-Function/1
  S-Function/1 -> Demux/1
  Demux/1 -> Outport3/1, Add/2, To Workspace/1, Scope/1  "x_s"
  Demux/2 -> Outport4/1, Add1/2, To Workspace1/1, Scope/2  "y_s"
  Demux/3 -> To Workspace4/1, Outport1/1, Sin1/1, Sin/1, Scope/3  "psi"
  In1/1 -> Bicycle Kinematic Model/1, Mux/1
  In3/1 -> Degrees to Radians/1, Mux/3
  Bicycle Kinematic Model/1 -> Demux1/1
  Outport/1 -> Mux/2
  Demux1/1 -> XY Graphd/1  "x"
  Demux1/2 -> XY Graphd/2  "y"
  Degrees to Radians/1 -> Bicycle Kinematic Model/2
  In4/1 -> Mux/4
  In5/1 -> Mux/5
  In6/1 -> Mux/6
  Demux/4 -> Outport2/1, Scope/4  "psi_dot_dot_s"
  Inport1/1 -> Mux/8
  Inport/1 -> Mux/7
  Gain/1 -> Add/1
  Sin1/1 -> Gain2/1
  Sin/1 -> Gain/1
  Gain2/1 -> Add1/1
  Add1/1 -> Kognitiv1/2, To Workspace3/1, Scope1/1, y_s/1  "y_st"
  Add/1 -> Kognitiv1/1, To Workspace2/1, x_s/1  "x_st"

== system Fahrzeugmodell/Positionsbestimmung/Sensormodelle ==
  x4=psi_dot2 : Inport
  x4=psi_dot1 : Inport  Port=2
  x4=psi_ot : Inport  Port=3
  Scope3 : Scope  NumInputPorts=4
  Sensormodell : Subsystem  TreatAsAtomicUnit=on  SystemSampleTime=0.01
  v_x : Outport
  Outport : Outport  Port=2
  Out3 : Outport  Port=3
  wires:
  x4=psi_dot2/1 -> Sensormodell/1(x4=psi_dot2)
  Sensormodell/1(Out1) -> Out3/1, Scope3/1
  Sensormodell/2(Outport) -> Scope3/2, Outport/1
  x4=psi_ot/1 -> Sensormodell/2(x4=psi_dot)
  Sensormodell/4(Out3) -> Scope3/4
  Sensormodell/3(v_x) -> v_x/1, Scope3/3
  x4=psi_dot1/1 -> Sensormodell/3(x4=psi_dot1)

== system Fahrzeugmodell/Trigger/Subsystem1 ==
  In1 : Inport
  In2 : Inport  Port=2
  In3 : Inport  Port=3
  In4 : Inport  Port=4
  Abs : Abs
  Compare To Constant : simulink/Logic and Bit Operations/Compare To Constant  relop=>=  const=0.1  OutDataTypeStr=boolean
  Lookup Table Dynamic : simulink/Lookup Tables/Lookup Table Dynamic  LookUpMeth=Interpolation-Use End Values  OutDataType=fixdt('double')  OutScaling=[]  OutputDataTypeScalingMode=Specify via dialog  OutDataTypeStr=double  DoSatur=off
  Scope : Scope
  Subtract : Sum  Inputs=+-
  To Workspace : ToWorkspace  VariableName=y_soll  SaveFormat=Timeseries  SampleTime=-1
  y : Outport
  wires:
  Compare To Constant/1 -> y/1, Scope/1  "Ja/nein"
  Subtract/1 -> Abs/1
  Abs/1 -> Compare To Constant/1
  In1/1 -> Lookup Table Dynamic/1
  Lookup Table Dynamic/1 -> Subtract/1
  In3/1 -> Lookup Table Dynamic/3, To Workspace/1
  In4/1 -> Subtract/2
  In2/1 -> Lookup Table Dynamic/2

== system Fahrzeugmodell/Trigger/Subsystem2 ==
  R : Inport
  Ja/Nein : Inport  Port=2
  AND1 : Logic  IconShape=distinctive  AllPortsSameDT=off  OutDataTypeStr=boolean
  Clock1 : Clock
  Constant : Constant  Value=0
  Data Type Conversion1 : DataTypeConversion  OutDataTypeStr=boolean
  Equal : RelationalOperator  Operator===  OutDataTypeStr=boolean  RndMeth=Simplest
  OR : Logic  Operator=OR  IconShape=distinctive  AllPortsSameDT=off  OutDataTypeStr=boolean
  Rate Transition1 : RateTransition  OutPortSampleTime=1
  S-R Flip-Flop1 : simulink_extras/Flip Flops/S-R Flip-Flop  initial_condition=0
  Scope10 : Scope
  !Q : Outport
  Out2 : Outport  Port=2
  wires:
  Rate Transition1/1 -> AND1/1  "Laterale Abweichung"
  OR/1 -> Out2/1, Scope10/1
  Data Type Conversion1/1 -> S-R Flip-Flop1/1
  Equal/1 -> OR/2
  Clock1/1 -> Equal/1
  S-R Flip-Flop1/1 -> AND1/2
  [C1] -> Data Type Conversion1/1
  AND1/1 -> OR/1
  Constant/1 -> Equal/2
  Ja/Nein/1 -> Rate Transition1/1
  S-R Flip-Flop1/2 -> !Q/1
  R/1 -> S-R Flip-Flop1/2

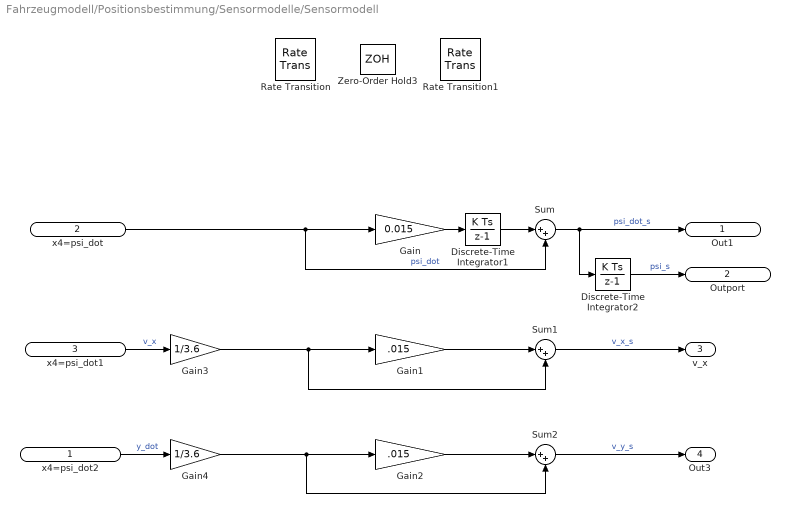
== system Fahrzeugmodell/Positionsbestimmung/Sensormodelle/Sensormodell ==
  x4=psi_dot2 : Inport
  x4=psi_dot : Inport  Port=2
  x4=psi_dot1 : Inport  Port=3
  Discrete-Time Integrator1 : DiscreteIntegrator  SampleTime=0.01  ICPrevOutput=DiscIntNeverNeededParam  ICPrevScaledInput=DiscIntNeverNeededParam
  Discrete-Time Integrator2 : DiscreteIntegrator  SampleTime=0.01  ICPrevOutput=DiscIntNeverNeededParam  ICPrevScaledInput=DiscIntNeverNeededParam
  Gain : Gain  Gain=0.015
  Gain1 : Gain  Gain=.015
  Gain2 : Gain  Gain=.015
  Gain3 : Gain  Gain=1/3.6
  Gain4 : Gain  Gain=1/3.6
  Rate Transition : RateTransition
  Rate Transition1 : RateTransition
  Sum : Sum  Inputs=|++
  Sum1 : Sum  Inputs=|++
  Sum2 : Sum  Inputs=|++
  Zero-Order Hold3 : ZeroOrderHold  SampleTime=0.01
  Out1 : Outport
  Outport : Outport  Port=2
  v_x : Outport  Port=3
  Out3 : Outport  Port=4
  wires:
  Gain/1 -> Discrete-Time Integrator1/1
  Discrete-Time Integrator1/1 -> Sum/1
  Sum/1 -> Discrete-Time Integrator2/1, Out1/1  "psi_dot_s"
  x4=psi_dot/1 -> Sum/2, Gain/1  "psi_dot"
  Gain3/1 -> Sum1/2, Gain1/1
  Sum1/1 -> v_x/1  "v_x_s"
  Gain1/1 -> Sum1/1
  Discrete-Time Integrator2/1 -> Outport/1  "psi_s"
  Gain2/1 -> Sum2/1
  Sum2/1 -> Out3/1  "v_y_s"
  x4=psi_dot2/1 -> Gain4/1  "y_dot"
  x4=psi_dot1/1 -> Gain3/1  "v_x"
  Gain4/1 -> Sum2/2, Gain2/1

== matlab function Fahrzeugmodell/MATLAB Function1 ==
  data: t input; T output
function T = fcn(t)
x=floor(t/2);
T=t-x*2;

== matlab function Fahrzeugmodell/MATLAB Function2 ==
  data: x_soll input; delta_soll output; x_ist input; delta_soll input
function delta_soll = fcn(x_soll, x_ist, delta_soll)
for i=1:1:100
    e_alt=1;
    e_ist= abs(x_soll(i)-x_ist);
    
    if e_ist<e_alt
        e_alt=e_ist;
        delta_v=delta_soll(i);
    end
end

== matlab function Fahrzeugmodell/Positionsbestimmung/MATLAB Function2 ==
  data: delta_v input; delta_r output; delta_l output
function [delta_r,delta_l] = fcn(delta_v)

a   = 1.25;      %Abstand Vorderachse zum Schwerpunkt m   
b   = 1.35;      %Abstand Hinterachse zum Schwerpunkt m

ab=1.788;        % Auto Bereite m
av=0.8;          % Voderachse zum Autovorderseite
bh=0.8;          % Hintenachse zum Autohintenseite


R=(a+b)/tan(delta_v); % Wendekreisradius auf dem Einspurmdell
delta_r=atan((a+b)/(R-ab/2)); % Wendekreisradius des rechten Reifens 
delta_l=atan((a+b)/(R+ab/2)); % Wendekreisradius des linken Reifens

== matlab function Fahrzeugmodell/Positionsbestimmung/MATLAB Function3 ==
  data: x_s input; x12 output; y_s input; psi_s input; delta_r input; delta_l input
function x12 = fcn(x_s,y_s,psi_s,delta_r,delta_l)

a   = 1.25;      %Abstand Vorderachse zum Schwerpunkt m   
b   = 1.35;      %Abstand Hinterachse zum Schwerpunkt m

ab=1.788;        % Auto Bereite m
av=0.8;          % Voderachse zum Autovorderseite
bh=0.8;          % Hintenachse zum Autohintenseite


Rz1=[cos(psi_s) -sin(psi_s)  x_s;
     sin(psi_s) cos(psi_s)   y_s;
     0          0            1  ;];
RzVL=[cos(delta_l) -sin(delta_l) a;
      sin(delta_l)  cos(delta_l) ab/2;
      0             0            1;];
XVL1=[0.4 0.15 1];
XVL0=Rz1*RzVL*XVL1';
x12=XVL0(1);

plot(x_s,x12,'ko');
hold on;

== matlab function Fahrzeugmodell/Positionsbestimmung/MATLAB Function4 ==
  data: x_M input; m1 output; m2 output; m3 output; y_M input; psi_M input; X_det output
function [m1,m2,m3,X_det]= Detektion1(x_M,y_M,psi_M)
% Abstände zwischen jeweils zwei Tags aufeinander liegen
d=0.1414;
% erste Reihe von E-Tags
n=linspace(1,17,17);
X1=zeros(35,2);
X1(2*n-1,1)=5;
X1(2*n,1)=5+d;
X1(2*n-1,2)=(2*n-1)*d;
X1(2*n,2)=2*n*d;
% zweite Reihe von E-Tags
X2=zeros(35,2);
X2(2*n-1,1)=10;
X2(2*n,1)=10+d;
X2(2*n-1,2)=(2*n-1)*d;
X2(2*n,2)=2*n*d;
% Homogene Transformationsmatrix auf dem Schwerpunkt
Hz1=[cos(psi_M) -sin(psi_M)   x_M;
     sin(psi_M)  cos(psi_M)   y_M;
     0           0            1  ;];
% Homogene Transformationsmatrix von Schwerpunkt auf Antenne
HtA=[1          0              1.35 ;
     0          1              0 ;
     0          0              1 ;];
% Detektionsquerschnitt der Antenne
XA1=[-0.1 -0.1 1];  
XA2=[0.1  -0.1 1];  
XA3=[0.1   0.1 1];  
XA4=[-0.1  0.1 1]; 
% Inverse Umrechnung der Koordinate der Antenne auf Weltkoordinate
XA1=Hz1*HtA*XA1.';
XA2=Hz1*HtA*XA2.';
XA3=Hz1*HtA*XA3.';
XA4=Hz1*HtA*XA4.';
% Anordnung vier Ecken
xA=[XA1(1) XA2(1) XA3(1) XA4(1) XA1(1)];
yA=[XA1(2) XA2(2) XA3(2) XA4(2) XA1(2)];
% Intialisierung der Detektionssignale
m1=0;
m2=0;
m3=0;
% Relative Koordinate der detektierten E-Tags in Antennekoordinate
% (Deklaration)
X_det=[0;
       0;
       1];
% 35 E- Tags verteilen sich innerhalb 5 Meter
for n=1:1:35
    in1=inpolygon(X1(n,1),X1(n,2),xA,yA);
    in2=inpolygon(X2(n,1),X2(n,2),xA,yA);
    in3=inpolygon(14,2.5,xA,yA);
    if in1
        m1=double(in1);
        x_det=X1(n,1);
        y_det=X1(n,2);
        X_det=[x_det;
               y_det;
                    1];
        X_det=inv(Hz1)*inv(HtA)*X_det;
        break;
    elseif in2
        m2=double(in2);
        x_det=X2(n,1);
        y_det=X2(n,2);
        X_det=[x_det;
               y_det;
                    1];
        X_det=inv(Hz1)*inv(HtA)*X_det;
        break;
    elseif in3
        m3=double(in3);
        x_det=14;
        y_det=2.5;
        X_det=[x_det;
            y_det;
            1];
        X_det=inv(Hz1)*inv(HtA)*X_det;
        break;
    end
end

== matlab function Fahrzeugmodell/Bahnplanung/Subsystem/aus BA_Li ==
  data: xs input; x_soll output; ys input; dys input; xe input; ye input; dye input; kappa_max input; y_soll output; Kappa_soll output
function [x_soll,y_soll,Kappa_soll] = Bezier4(xs,ys,dys,xe,ye,dye,kappa_max)
% 
x_soll = zeros(101,1);
y_soll = zeros(101,1);
Kappa_soll = zeros(101,1);

coder.extrinsic('Bezier');

% 2DOF

[x_soll,y_soll,Kappa_soll]=Bezier(xs,ys,dys,xe,ye,dye,kappa_max);



% 6DOF
% x_soll = zeros(50,1);
% y_soll = zeros(50,1);
% Kappa_soll = zeros(50,1);
% 
% coder.extrinsic('Bezier1');
% 
% [x_soll,y_soll,Kappa_soll]=Bezier1(xs,ys,dys,xe,ye,dye,kappa_max);

== matlab function Fahrzeugmodell/Positionsbestimmung/MATLAB Function ==
  data: x_M input; M output; y_M input; M1 output; M2 output
function [M, M1, M2] = Detektion(x_M,y_M)

xv= [5 5.4 5.4 5 5 NaN 5.4 5.8 5.8 5.4 5.4 NaN ...
    5 5.4 5.4 5 5 NaN 5.4 5.8 5.8 5.4 5.4 NaN ...
    5 5.4 5.4 5 5 NaN 5.4 5.8 5.8 5.4 5.4 NaN ...
    5 5.4 5.4 5 5 NaN 5.4 5.8 5.8 5.4 5.4 NaN ...
    5 5.4 5.4 5 5 NaN 5.4 5.8 5.8 5.4 5.4 NaN ...
    5 5.4 5.4 5 5 NaN 5.4 5.8 5.8 5.4 5.4 NaN];

xv1=[10 10.4 10.4 10 10 NaN 10.4 10.8 10.8 10.4 10.4 NaN...
    10 10.4 10.4 10 10 NaN 10.4 10.8 10.8 10.4 10.4 NaN...
    10 10.4 10.4 10 10 NaN 10.4 10.8 10.8 10.4 10.4 NaN...
    10 10.4 10.4 10 10 NaN 10.4 10.8 10.8 10.4 10.4 NaN...
    10 10.4 10.4 10 10 NaN 10.4 10.8 10.8 10.4 10.4 NaN...
    10 10.4 10.4 10 10 NaN 10.4 10.8 10.8 10.4 10.4 NaN];
xv2=[13.8 14.2 14.2 13.8 13.8 NaN]; %X-Verbotener Bereich

yv= [0  0   0.4 0.4 0   NaN 0.4 0.4 0.8 0.8 0.4 NaN ...
    0.8 0.8 1.2 1.2 0.8 NaN 1.2 1.2 1.6 1.6 1.2 NaN ...
    1.6 1.6 2.0 2.0 1.6 NaN 2.0 2.0 2.4 2.4 2.0 NaN ...
    2.4 2.4 2.8 2.8 2.4 NaN 2.8 2.8 3.2 3.2 2.8 NaN ...
    3.2 3.2 3.6 3.6 3.2 NaN 3.6 3.6 4.0 4.0 3.6 NaN ...
    4.0 4.0 4.4 4.4 4.0 NaN 4.4 4.4 4.8 4.8 4.4 NaN];

yv1=[0   0   0.4 0.4 0   NaN 0.4 0.4 0.8 0.8 0.4 NaN ...
    0.8 0.8 1.2 1.2 0.8 NaN 1.2 1.2 1.6 1.6 1.2 NaN ...
    1.6 1.6 2.0 2.0 1.6 NaN 2.0 2.0 2.4 2.4 2.0 NaN ...
    2.4 2.4 2.8 2.8 2.4 NaN 2.8 2.8 3.2 3.2 2.8 NaN ...
    3.2 3.2 3.6 3.6 3.2 NaN 3.6 3.6 4.0 4.0 3.6 NaN ...
    4.0 4.0 4.4 4.4 4.0 NaN 4.4 4.4 4.8 4.8 4.4 NaN];
yv2=[2.2 2.2 2.6 2.6 2.2 NaN];% Y-Verbotener Bereich


in=inpolygon(x_M,y_M,xv,yv);
in1=inpolygon(x_M,y_M,xv1,yv1);
in2=inpolygon(x_M,y_M,xv2,yv2);
M= double(in);
M1= double(in1);
M2= double(in2);

== matlab function Fahrzeugmodell/Laengsdynamik/MATLAB Function ==
  data: v_x input; P output; v_x_dot input; v_y input; psi_dot input
function P  = Verifizierung_Laengsdynamik(v_x,v_x_dot,v_y,psi_dot)
%% Parameter der Längsdynamik deklarieren
m   = 1359.8;       %Masse Fahrzeugs                     kg
c_w = 0.34;         %Luftwiderstandbeiwert           
roh = 1.225;        %Luftdichte bei 25 °C                kg/m^3
A_f = 1.6 + 0.00056*(m-765);        %Querfläche        m^2
f_r  = 0.015;        %Rollwiderstandbeiwert
g   = 9.81;         %Erdebeschleunigung

%% Umrechnen der Vorgabe der Leistung
% P = 1/2*c_w*roh*A_f*v^3+f_r*m*g*v; %% Leistung

P=m*(v_x_dot-v_y*psi_dot)*v_x+1/2*c_w*roh*A_f*v_x^2+m*g*f_r*v_x;

end

== matlab function Fahrzeugmodell/Bahnplanung/Subsystem/aus doi: 10.1177//1464419320924196. Algorithm 1 ==
  data: Fehler output; x0 input; kappa1 output; y0 input; dy0 input; d2y0 input; xf input; yf input; dyf input; d2yf input; kappa_M input; xs output; ys output; kappa_max output
function [ Fehler,kappa1,xs,ys,kappa_max]   = Bahnplanung(x0,y0,dy0,d2y0,xf,yf,dyf,d2yf,kappa_M)
%% Algorithmus 1, Optimierung der konventionellen Methode
% Deklaration



%% Positionsvorgabe
% y0=2;
% dy0=0.2;
% d2y0=0;
% yf=3;
% dyf=0;
% d2yf=0;

%% 
% Randbedingungsmatrix nach der Positionsvorgabe
Gamma=[0, dy0, d2y0, yf-y0, dyf, d2yf];

% Vorgabe der max. Krümmung
% kappa_M = 0.175;
% Initialwert der Länge zur Optimierung
L=2/kappa_M;
s_l= xf-x0;
Fehler=0;
%% Ergondisch entscheiden bis die max. Krümmung kleiner als die Vorgabe
while 1
    s=s_l+max(floor(L)-s_l,0);
    
    xi=linspace(0,1,s);
%     xiq=0:0.01:1;
    a5_stern=6*Gamma(4)-3*Gamma(2)*L-3*Gamma(5)*L-Gamma(3)*L^2/2+Gamma(6)*L^2/2;
    a4_stern=8*Gamma(2)*L-15*Gamma(4)+7*Gamma(5)*L+3*Gamma(3)*L^2/2-Gamma(6)*L^2;
    a3_stern=10*Gamma(4)-6*Gamma(2)*L-4*Gamma(5)*L-3*Gamma(3)*L^2/2+Gamma(6)*L^2/2;
    a2_stern=Gamma(3)*L^2/2;
    a1_stern=Gamma(2)*L;
    a0_stern=0;
    
    y=a5_stern*xi.^5+a4_stern*xi.^4+a3_stern*xi.^3+a2_stern*xi.^2+a1_stern*xi+0;
%     vy1=interp1(xi,y,xiq,'spline');
%     ys=vy1*(yf-y0)/yf+y0;
%     ys=vy1+y0;
    dy=1/L*(5*a5_stern*xi.^4+4*a4_stern*xi.^3+3*a3_stern*xi.^2+a2_stern*xi+a1_stern);
    d2y=1/L/L*(20*a5_stern*xi.^3+12*a4_stern*xi.^2+6*a3_stern*xi+2*a2_stern);
    kappa=d2y./power((1+dy.^2),1.5);
%     kappa1=interp1(xi,kappa,xiq,'spline')/3;
    kappa_max=max(abs(kappa));
%     
    if kappa_max<0.174
        
        e=1e-4;
%         Fehler=1;
%         break;
    else
        e=1/kappa_M-1/kappa_max;
    end
    
    if abs(e)< 1e-3
        L_opt=L;
%         Fehler=0;
        break;
    else
        L=L+e;
        continue;
    end
end
% kappa_ers=zeros(1,101);
xiq=0:0.01:1;
xs=linspace(x0,xf,length(xiq));
vy1=interp1(xi,y,xiq,'spline');
ys=vy1+y0;
kappa1=interp1(xi,kappa,xiq,'spline');

if kappa_max>0.175
    Fehler=1;
  
end

% if Fehler==0
%     kappa_ers=kappa1;
%     
% end

%%
% coder.varsize('ys', [Inf 1],[1 0]);
% coder.varsize('s', [Inf 1],[1 0]);

% kappa_s=kappa(1);
% xs=linspace(x0,xf,s*10);
% subplot(2,1,1);
% 
% 
% plot(xv,yv);
% hold on;
% 
% rectangle('Position',[0 0 15 5]);
% axis([-1 18 0 5]);
% hold on;
% 
% plot(x0,y0,'b--o');
% hold on;
% 
% plot(xs,ys);
% ylabel('$lateral_\mathrm{y}$ in m','Interpreter','latex');
% xlabel('$longitudinal_\mathrm{x}$ in m','Interpreter','latex');
% axis equal;
% hold on;

% subplot(2,1,2);
% plot(s,kappa);
% ylabel('$Kruemmung$ in  $m^{-1}$ ','Interpreter','latex');
% xlabel('$longitudinal_\mathrm{x}$ in m','Interpreter','latex');
% hold on;

== matlab function Fahrzeugmodell/Positionsbestimmung/MATLAB Function1 ==
  data: x_st input; y_st input; x_s input; y_s input; psi_s input; x_soll input; y_soll input; delta_r input; delta_l input
function Fahranimation(x_st, y_st,x_s, y_s, psi_s,x_soll,y_soll, delta_r, delta_l)
coder.extrinsic('ZweiDFahranimation');

ZweiDFahranimation(x_st, y_st,x_s, y_s, psi_s,x_soll,y_soll, delta_r, delta_l)

== matlab function Fahrzeugmodell/MATLAB Function ==
  data: delta_soll input; delta_v output; t input
function delta_v = fcn(delta_soll, t)

% ts=t*50+10;
ts=t/0.066+1;

delta_v=delta_soll(ts);

== matlab function Fahrzeugmodell/Bahnplanung/Subsystem/aus BA_Malert ==
  data: x0 input; kappa output; y0 input; dy0 input; d2y0 input; x1 input; y1 input; dy1 input; d2y1 input; kappa_M input; x output; y output; abbiegen output; s output
function  [kappa,x,y,abbiegen,s]   = Bahnplanung1(x0,y0,dy0,d2y0,x1,y1,dy1,d2y1,kappa_M)

%%
% Start- und Endposition
% P0 = [x0;y0;dy0;d2y0]; % Startpunkt
% P1 = [xf;yf;dyf;d2yf]; % Zielpunkt

% Ermitteln der Koeffizienten für Polynom 5. Ordnung
A5 = [1 x0 (x0)^2 (x0)^3    (x0)^4     (x0)^5;
      1 x1 (x1)^2 (x1)^3    (x1)^4     (x1)^5;
      0 1   2*x0  3*(x0)^2 4*(x0)^3   5*(x0)^4;
      0 1   2*x1  3*(x1)^2 4*(x1)^3   5*(x1)^4;
      0 0    2     6*x0    12*(x0)^2  20*(x0)^3;
      0 0    2     6*x1    12*(x1)^2  20*(x1)^3]; % Matrix des linearen Gleichungssystems
  
b5 = [y0; y1; dy0; dy1; d2y0; d2y1];               % Ergebnisvektor
a5 = A5 \ b5;                            % Koeffizientenvektor berechnenA5

a50 = a5(1); 
a51 = a5(2); 
a52 = a5(3); 
a53 = a5(4); 
a54 = a5(5); 
a55 = a5(6);   % Hilfsvariabeln

% Überprüfung des maximal möglichen Lenkwinkels

x = linspace(x0,x1,100);
y  = a50+a51*x+a52*x.^2+a53*x.^3+a54*x.^4+a55*x.^5;    % f(x) berechnen x Koordinate
dy = a51+a52*2*x+a53*3*x.^2+a54*4*x.^3+a55*5*x.^4;   % f'(x) berechnen  Gierwinkel 
d2y = a52*2+a53*6*x+a54*12*x.^2+a55*20*x.^3;         % f''(x) berechnen  Gierrate
% kappa = d2y./(1+dy.^2).^(3/2);                              % Bahnkrümmung bestimmen
kappa=d2y./power((1+dy.^2),1.5);
kappa_s=kappa(2);

    if kappa_M>max(abs(kappa))
        abbiegen=1;
        
    else
        abbiegen=0;
        
    end


%% zurückgelegte Strecke berechnen
s=0;
for i = 1:(length(x)-1)
    s = s + sqrt((x(i+1)-x(i))^2+(y(i+1)-y(i))^2);
end
struct
%%
% Trajektorienplanung

% Eingabe der Anfangsbedingung
v0=2;
a0=0;
t=10;


% Matrixrechnung
V0=[0,v0];                    % Anfangsbedingung bei t=0   v=v0
V1=[t,0];                     % Endbedingung     bei t=t   v=0
t0=V0(1);v0=V0(2); t1=V1(1); v1=V0(2);

% Ermitteln der Koeffizienten für Polynom 5. Ordnung
% Durch Interpolation für Geschwindigkeit und Beschleunigung
M5=[1 t0 t0^2 t0^3   t0^4     t0^5;
    0 1  2*t0 3*t0^2 4*t0^3   5*t0^4;  
    0 0  2    6*t0   12*t0^2  20*t0^3;
    1 t1 t1^2 t1^3   t1^4     t1^5;
    0 1  2*t1 3*t1^2 4*t1^3   5*t1^4;
    0 0  2    6*t1   12*t1^2  20*t1^3;];   % Matrix des linearen Systems

n5=[0;v0; a0; s; 0; 0;];            % Ergebnisvektor

m5=M5 \ n5;                    %Koeffizientenvektor

m50=m5(1);
m51=m5(2);
m52=m5(3);
m53=m5(4);
m54=m5(5);                     % Termen des Koeffizientenvektors
m55=m5(6);

T=[0:0.01:t];                  % regelte Einparkzeit

S=m50+m51*T+m52*T.^2+m53*T.^3+m54*T.^4+m55*T.^5;

v=m51+2*m52*T+3*m53*T.^2+4*m54*T.^3+5*m55*T.^4;  % Geschwindigkeit berechnen

a=2*m52+6*m53*T+12*m54*T.^2+20*m55*T.^3;          % Beschleunigung berechnen


%% Grafische Darstellung Trajektorienplanung
% figure('Name','Streckenprofil');                          % Wegstreckenprofil
% plot(T,S,'Linestyle','-','color',[0 0.9 0]); 
% ylabel('$Wegstrecke$ in m','Interpreter','latex');
% xlabel('$Zeit$ in s','Interpreter','latex');
% 
% figure('Name','Geschwindigkeitsprofil');                  % Geschwindigkeitsprofil
% plot(T,v,'Linestyle','-','color',[0 0.3 0]); 
% ylabel('$Geschwindigkeit$ in m/s','Interpreter','latex');
% xlabel('$Zeit$ in s','Interpreter','latex');
% 
% figure('Name','Beschleunigungsprofil');                   % Beschleunigungsprofil
% plot(T,a,'Linestyle','-','color',[0 0.7 1]);  
% ylabel('$Beschleunigung$ in $m/s^2$','Interpreter','latex');
% xlabel('$Zeit$ in s','Interpreter','latex');
% hold on;

% plot(x,kappa,'Linestyle','-','color',[0 0.7 1]);  
% hold on;
%% Grafische Darstellung Bahnplanung
% figure('Name','Bahnplanung');
% plot(x,y,'Linestyle','-','color',[0 0.6 0]);                % Bahn
% 
% ylabel('$lateral_\mathrm{y}$ in m','Interpreter','latex');
% xlabel('$longitudinal_\mathrm{x}$ in m','Interpreter','latex');
% hold on;
% xlim([0 10]);
% ylim([-10 0]);
% axis equal;

% plot(x,abbiegen);
% hold on;
%
